simulink library "rov_design_analysis"  (Simulink 6.0)
settings: Solver=ode45  SolverMode=SingleTasking  StartTime=0.0  StopTime=10.0  RelTol=1e-3
undefined symbols (not defined in the file or in its folder): amp, At, B, Bt, Ct, cycles, D, den, DL, Do, DQ, DQL, freq, frtest, I, L, m, M, Ma, magnitude, MaU, Mt, nmiss, num, phase, rg, sigbuilder_block, slcm, T, W, xb, xg, Xudot, yb, yg, Yvdot, zb, zg, Zwdot
libraries: simulink_extras x32, simulink x27, rov_design_analysis x15, marine_gnc x10, dspmtrx2 x6, dspstat3 x4
(part 8 of 9)

== system rov_design_analysis/ROV Controller /Nonlinear-Sliding-Mode Cascaded  Controller - 6 DoF/Body-fixed to Earth_fixed Transformation3/Transformation matrix T/Row3 of R ==
  translational body velocity : Inport  Port=1  LatchInput=off
  angular position : Inport  Port=2  LatchInput=off
  -cZ.sX+sY.sZ.cX : Fcn  Expr=-cos(u[3])*sin(u[1]) + sin(u[2])*sin(u[3])*cos(u[1])
  Dot Product1 : Subsystem  mask(Dot Product){}
      mask help:
      | Inner (dot) product.
      | y=sum(u1.*u2)
      mask init:
      | t=(0:.1:2*pi)';
      | x=cos(t);
      | y=sin(t);
      mask Help: Computes the inner (dot) product of the inputs: sum(u1.*u2).  The inputs are vectors of the same length. Output is a scalar.
      mask Display: plot(0,0,1,1,x*[0.025 0.07]+0.5,y*[0.025 0.07]+0.5)
  Mux1 : Mux  Inputs=3
  cY.cX : Fcn  Expr=cos(u[2])*cos(u[1])
  sZ.sX+cZ.cX.sY : Fcn  Expr=sin(u[3])*sin(u[1]) + cos(u[3])*cos(u[1])*sin(u[2])
  translational earth velocity (row 3) : Outport  InitialOutput=0
  wires:
  Dot Product1/1(out_1) -> translational earth velocity (row 3)/1
  translational body velocity/1 -> Dot Product1/2(in_2)
  Mux1/1 -> Dot Product1/1(in_1)
  cY.cX/1 -> Mux1/3
  -cZ.sX+sY.sZ.cX/1 -> Mux1/2
  sZ.sX+cZ.cX.sY/1 -> Mux1/1
  angular position/1 -> cY.cX/1, -cZ.sX+sY.sZ.cX/1, sZ.sX+cZ.cX.sY/1

== system rov_design_analysis/ROV Controller /P-Decoupled  Cascaded loop Controller  - 6 DoF/Body-fixed to Earth_fixed Transformation1/Transformation matrix R/Row1 of T ==
  angular body  velocity : Inport  Port=1  LatchInput=off
  angular position : Inport  Port=2  LatchInput=off
  0 : Fcn  Expr=0
  1 : Fcn  Expr=1
  2 : Fcn  Expr=0
  Dot Product1 : Subsystem  mask(Dot Product){}
      mask help:
      | Inner (dot) product.
      | y=sum(u1.*u2)
      mask init:
      | t=(0:.1:2*pi)';
      | x=cos(t);
      | y=sin(t);
      mask Help: Computes the inner (dot) product of the inputs: sum(u1.*u2).  The inputs are vectors of the same length. Output is a scalar.
      mask Display: plot(0,0,1,1,x*[0.025 0.07]+0.5,y*[0.025 0.07]+0.5)
  Mux1 : Mux  Inputs=3
  angular earth velocity (row 1) : Outport  InitialOutput=0
  wires:
  angular position/1 -> 1/1, 0/1, 2/1
  1/1 -> Mux1/1
  0/1 -> Mux1/2
  2/1 -> Mux1/3
  Mux1/1 -> Dot Product1/1(in_1)
  angular body  velocity/1 -> Dot Product1/2(in_2)
  Dot Product1/1(out_1) -> angular earth velocity (row 1)/1

== system rov_design_analysis/ROV Controller /P-Decoupled  Cascaded loop Controller  - 6 DoF/Body-fixed to Earth_fixed Transformation1/Transformation matrix R/Row2 of T ==
  "angular body velocity " : Inport  Port=1  LatchInput=off
  angular position : Inport  Port=2  LatchInput=off
  Dot Product1 : Subsystem  mask(Dot Product){}
      mask help:
      | Inner (dot) product.
      | y=sum(u1.*u2)
      mask init:
      | t=(0:.1:2*pi)';
      | x=cos(t);
      | y=sin(t);
      mask Help: Computes the inner (dot) product of the inputs: sum(u1.*u2).  The inputs are vectors of the same length. Output is a scalar.
      mask Display: plot(0,0,1,1,x*[0.025 0.07]+0.5,y*[0.025 0.07]+0.5)
  Mux1 : Mux  Inputs=3
  cX : Fcn  Expr=cos(u[1])
  sX.tY : Fcn  Expr=sin(u[1])*tan(u[2])
  sX/cY : Fcn  Expr=sin(u[1])/cos(u[2])
  angular earth velocity (row 2) : Outport  InitialOutput=0
  wires:
  angular position/1 -> sX.tY/1, cX/1, sX/cY/1
  sX.tY/1 -> Mux1/1
  cX/1 -> Mux1/2
  sX/cY/1 -> Mux1/3
  Mux1/1 -> Dot Product1/1(in_1)
  "angular body velocity "/1 -> Dot Product1/2(in_2)
  Dot Product1/1(out_1) -> angular earth velocity (row 2)/1

== system rov_design_analysis/ROV Controller /P-Decoupled  Cascaded loop Controller  - 6 DoF/Body-fixed to Earth_fixed Transformation1/Transformation matrix R/Row3 of T ==
  "angular body velocity " : Inport  Port=1  LatchInput=off
  angular position : Inport  Port=2  LatchInput=off
  -sX : Fcn  Expr=-sin(u[1])
  Dot Product1 : Subsystem  mask(Dot Product){}
      mask help:
      | Inner (dot) product.
      | y=sum(u1.*u2)
      mask init:
      | t=(0:.1:2*pi)';
      | x=cos(t);
      | y=sin(t);
      mask Help: Computes the inner (dot) product of the inputs: sum(u1.*u2).  The inputs are vectors of the same length. Output is a scalar.
      mask Display: plot(0,0,1,1,x*[0.025 0.07]+0.5,y*[0.025 0.07]+0.5)
  Mux1 : Mux  Inputs=3
  cX.tY : Fcn  Expr=cos(u[1])*tan(u[2])
  cX/cY : Fcn  Expr=cos(u[1])/cos(u[2])
  angular earth velocity (row 3) : Outport  InitialOutput=0
  wires:
  angular position/1 -> cX.tY/1, -sX/1, cX/cY/1
  cX.tY/1 -> Mux1/1
  -sX/1 -> Mux1/2
  cX/cY/1 -> Mux1/3
  Mux1/1 -> Dot Product1/1(in_1)
  "angular body velocity "/1 -> Dot Product1/2(in_2)
  Dot Product1/1(out_1) -> angular earth velocity (row 3)/1

== system rov_design_analysis/ROV Controller /P-Decoupled  Cascaded loop Controller  - 6 DoF/Body-fixed to Earth_fixed Transformation1/Transformation matrix T/Row1 of R ==
  translational body velocity : Inport  Port=1  LatchInput=off
  angular position : Inport  Port=2  LatchInput=off
  -sY : Fcn  Expr=-sin(u[2])
  Dot Product : Subsystem  mask(Dot Product){}
      mask help:
      | Inner (dot) product.
      | y=sum(u1.*u2)
      mask init:
      | t=(0:.1:2*pi)';
      | x=cos(t);
      | y=sin(t);
      mask Help: Computes the inner (dot) product of the inputs: sum(u1.*u2).  The inputs are vectors of the same length. Output is a scalar.
      mask Display: plot(0,0,1,1,x*[0.025 0.07]+0.5,y*[0.025 0.07]+0.5)
  Mux : Mux  Inputs=3
  cY.cZ : Fcn  Expr=cos(u[3]) * cos(u[2])
  cY.sZ : Fcn  Expr=sin(u[3]) * cos(u[2])
  translational earth velocity (row 1) : Outport  InitialOutput=0
  wires:
  angular position/1 -> cY.cZ/1, cY.sZ/1, -sY/1
  cY.cZ/1 -> Mux/1
  cY.sZ/1 -> Mux/2
  -sY/1 -> Mux/3
  Mux/1 -> Dot Product/1(in_1)
  translational body velocity/1 -> Dot Product/2(in_2)
  Dot Product/1(out_1) -> translational earth velocity (row 1)/1

== system rov_design_analysis/ROV Controller /P-Decoupled  Cascaded loop Controller  - 6 DoF/Body-fixed to Earth_fixed Transformation1/Transformation matrix T/Row2 of R ==
  translational body velocity : Inport  Port=1  LatchInput=off
  angular position : Inport  Port=2  LatchInput=off
  -sZ.cX+cZ.sY.sX : Fcn  Expr=-sin(u[3])*cos(u[1]) + cos(u[3])*sin(u[2])*sin(u[1])
  Dot Product1 : Subsystem  mask(Dot Product){}
      mask help:
      | Inner (dot) product.
      | y=sum(u1.*u2)
      mask init:
      | t=(0:.1:2*pi)';
      | x=cos(t);
      | y=sin(t);
      mask Help: Computes the inner (dot) product of the inputs: sum(u1.*u2).  The inputs are vectors of the same length. Output is a scalar.
      mask Display: plot(0,0,1,1,x*[0.025 0.07]+0.5,y*[0.025 0.07]+0.5)
  Mux1 : Mux  Inputs=3
  cY.sX : Fcn  Expr=cos(u[2])*sin(u[1])
  cZ.cX+sX.sY.sZ : Fcn  Expr=cos(u[3])*cos(u[1]) + sin(u[1])*sin(u[2])*sin(u[3])
  translational earth velocity (row 2) : Outport  InitialOutput=0
  wires:
  angular position/1 -> -sZ.cX+cZ.sY.sX/1, cZ.cX+sX.sY.sZ/1, cY.sX/1
  -sZ.cX+cZ.sY.sX/1 -> Mux1/1
  cZ.cX+sX.sY.sZ/1 -> Mux1/2
  cY.sX/1 -> Mux1/3
  Mux1/1 -> Dot Product1/1(in_1)
  translational body velocity/1 -> Dot Product1/2(in_2)
  Dot Product1/1(out_1) -> translational earth velocity (row 2)/1

== system rov_design_analysis/ROV Controller /P-Decoupled  Cascaded loop Controller  - 6 DoF/Body-fixed to Earth_fixed Transformation1/Transformation matrix T/Row3 of R ==
  translational body velocity : Inport  Port=1  LatchInput=off
  angular position : Inport  Port=2  LatchInput=off
  -cZ.sX+sY.sZ.cX : Fcn  Expr=-cos(u[3])*sin(u[1]) + sin(u[2])*sin(u[3])*cos(u[1])
  Dot Product1 : Subsystem  mask(Dot Product){}
      mask help:
      | Inner (dot) product.
      | y=sum(u1.*u2)
      mask init:
      | t=(0:.1:2*pi)';
      | x=cos(t);
      | y=sin(t);
      mask Help: Computes the inner (dot) product of the inputs: sum(u1.*u2).  The inputs are vectors of the same length. Output is a scalar.
      mask Display: plot(0,0,1,1,x*[0.025 0.07]+0.5,y*[0.025 0.07]+0.5)
  Mux1 : Mux  Inputs=3
  cY.cX : Fcn  Expr=cos(u[2])*cos(u[1])
  sZ.sX+cZ.cX.sY : Fcn  Expr=sin(u[3])*sin(u[1]) + cos(u[3])*cos(u[1])*sin(u[2])
  translational earth velocity (row 3) : Outport  InitialOutput=0
  wires:
  angular position/1 -> sZ.sX+cZ.cX.sY/1, -cZ.sX+sY.sZ.cX/1, cY.cX/1
  sZ.sX+cZ.cX.sY/1 -> Mux1/1
  -cZ.sX+sY.sZ.cX/1 -> Mux1/2
  cY.cX/1 -> Mux1/3
  Mux1/1 -> Dot Product1/1(in_1)
  translational body velocity/1 -> Dot Product1/2(in_2)
  Dot Product1/1(out_1) -> translational earth velocity (row 3)/1

== system rov_design_analysis/ROV Controller /P-Decoupled  Cascaded loop Controller  - 6 DoF/Body-fixed to Earth_fixed Transformation3/Transformation matrix R/Row1 of T ==
  angular body  velocity : Inport  Port=1  LatchInput=off
  angular position : Inport  Port=2  LatchInput=off
  0 : Fcn  Expr=0
  1 : Fcn  Expr=1
  2 : Fcn  Expr=0
  Dot Product1 : Subsystem  mask(Dot Product){}
      mask help:
      | Inner (dot) product.
      | y=sum(u1.*u2)
      mask init:
      | t=(0:.1:2*pi)';
      | x=cos(t);
      | y=sin(t);
      mask Help: Computes the inner (dot) product of the inputs: sum(u1.*u2).  The inputs are vectors of the same length. Output is a scalar.
      mask Display: plot(0,0,1,1,x*[0.025 0.07]+0.5,y*[0.025 0.07]+0.5)
  Mux1 : Mux  Inputs=3
  angular earth velocity (row 1) : Outport  InitialOutput=0
  wires:
  Dot Product1/1(out_1) -> angular earth velocity (row 1)/1
  angular body  velocity/1 -> Dot Product1/2(in_2)
  Mux1/1 -> Dot Product1/1(in_1)
  2/1 -> Mux1/3
  0/1 -> Mux1/2
  1/1 -> Mux1/1
  angular position/1 -> 2/1, 0/1, 1/1

== system rov_design_analysis/ROV Controller /P-Decoupled  Cascaded loop Controller  - 6 DoF/Body-fixed to Earth_fixed Transformation3/Transformation matrix R/Row2 of T ==
  "angular body velocity " : Inport  Port=1  LatchInput=off
  angular position : Inport  Port=2  LatchInput=off
  Dot Product1 : Subsystem  mask(Dot Product){}
      mask help:
      | Inner (dot) product.
      | y=sum(u1.*u2)
      mask init:
      | t=(0:.1:2*pi)';
      | x=cos(t);
      | y=sin(t);
      mask Help: Computes the inner (dot) product of the inputs: sum(u1.*u2).  The inputs are vectors of the same length. Output is a scalar.
      mask Display: plot(0,0,1,1,x*[0.025 0.07]+0.5,y*[0.025 0.07]+0.5)
  Mux1 : Mux  Inputs=3
  cX : Fcn  Expr=cos(u[1])
  sX.tY : Fcn  Expr=sin(u[1])*tan(u[2])
  sX/cY : Fcn  Expr=sin(u[1])/cos(u[2])
  angular earth velocity (row 2) : Outport  InitialOutput=0
  wires:
  Dot Product1/1(out_1) -> angular earth velocity (row 2)/1
  "angular body velocity "/1 -> Dot Product1/2(in_2)
  Mux1/1 -> Dot Product1/1(in_1)
  sX/cY/1 -> Mux1/3
  cX/1 -> Mux1/2
  sX.tY/1 -> Mux1/1
  angular position/1 -> sX/cY/1, cX/1, sX.tY/1

== system rov_design_analysis/ROV Controller /P-Decoupled  Cascaded loop Controller  - 6 DoF/Body-fixed to Earth_fixed Transformation3/Transformation matrix R/Row3 of T ==
  "angular body velocity " : Inport  Port=1  LatchInput=off
  angular position : Inport  Port=2  LatchInput=off
  -sX : Fcn  Expr=-sin(u[1])
  Dot Product1 : Subsystem  mask(Dot Product){}
      mask help:
      | Inner (dot) product.
      | y=sum(u1.*u2)
      mask init:
      | t=(0:.1:2*pi)';
      | x=cos(t);
      | y=sin(t);
      mask Help: Computes the inner (dot) product of the inputs: sum(u1.*u2).  The inputs are vectors of the same length. Output is a scalar.
      mask Display: plot(0,0,1,1,x*[0.025 0.07]+0.5,y*[0.025 0.07]+0.5)
  Mux1 : Mux  Inputs=3
  cX.tY : Fcn  Expr=cos(u[1])*tan(u[2])
  cX/cY : Fcn  Expr=cos(u[1])/cos(u[2])
  angular earth velocity (row 3) : Outport  InitialOutput=0
  wires:
  Dot Product1/1(out_1) -> angular earth velocity (row 3)/1
  "angular body velocity "/1 -> Dot Product1/2(in_2)
  Mux1/1 -> Dot Product1/1(in_1)
  cX/cY/1 -> Mux1/3
  -sX/1 -> Mux1/2
  cX.tY/1 -> Mux1/1
  angular position/1 -> cX/cY/1, -sX/1, cX.tY/1

== system rov_design_analysis/ROV Controller /P-Decoupled  Cascaded loop Controller  - 6 DoF/Body-fixed to Earth_fixed Transformation3/Transformation matrix T/Row1 of R ==
  translational body velocity : Inport  Port=1  LatchInput=off
  angular position : Inport  Port=2  LatchInput=off
  -sY : Fcn  Expr=-sin(u[2])
  Dot Product : Subsystem  mask(Dot Product){}
      mask help:
      | Inner (dot) product.
      | y=sum(u1.*u2)
      mask init:
      | t=(0:.1:2*pi)';
      | x=cos(t);
      | y=sin(t);
      mask Help: Computes the inner (dot) product of the inputs: sum(u1.*u2).  The inputs are vectors of the same length. Output is a scalar.
      mask Display: plot(0,0,1,1,x*[0.025 0.07]+0.5,y*[0.025 0.07]+0.5)
  Mux : Mux  Inputs=3
  cY.cZ : Fcn  Expr=cos(u[3]) * cos(u[2])
  cY.sZ : Fcn  Expr=sin(u[3]) * cos(u[2])
  translational earth velocity (row 1) : Outport  InitialOutput=0
  wires:
  Dot Product/1(out_1) -> translational earth velocity (row 1)/1
  translational body velocity/1 -> Dot Product/2(in_2)
  Mux/1 -> Dot Product/1(in_1)
  -sY/1 -> Mux/3
  cY.sZ/1 -> Mux/2
  cY.cZ/1 -> Mux/1
  angular position/1 -> -sY/1, cY.sZ/1, cY.cZ/1

== system rov_design_analysis/ROV Controller /P-Decoupled  Cascaded loop Controller  - 6 DoF/Body-fixed to Earth_fixed Transformation3/Transformation matrix T/Row2 of R ==
  translational body velocity : Inport  Port=1  LatchInput=off
  angular position : Inport  Port=2  LatchInput=off
  -sZ.cX+cZ.sY.sX : Fcn  Expr=-sin(u[3])*cos(u[1]) + cos(u[3])*sin(u[2])*sin(u[1])
  Dot Product1 : Subsystem  mask(Dot Product){}
      mask help:
      | Inner (dot) product.
      | y=sum(u1.*u2)
      mask init:
      | t=(0:.1:2*pi)';
      | x=cos(t);
      | y=sin(t);
      mask Help: Computes the inner (dot) product of the inputs: sum(u1.*u2).  The inputs are vectors of the same length. Output is a scalar.
      mask Display: plot(0,0,1,1,x*[0.025 0.07]+0.5,y*[0.025 0.07]+0.5)
  Mux1 : Mux  Inputs=3
  cY.sX : Fcn  Expr=cos(u[2])*sin(u[1])
  cZ.cX+sX.sY.sZ : Fcn  Expr=cos(u[3])*cos(u[1]) + sin(u[1])*sin(u[2])*sin(u[3])
  translational earth velocity (row 2) : Outport  InitialOutput=0
  wires:
  Dot Product1/1(out_1) -> translational earth velocity (row 2)/1
  translational body velocity/1 -> Dot Product1/2(in_2)
  Mux1/1 -> Dot Product1/1(in_1)
  cY.sX/1 -> Mux1/3
  cZ.cX+sX.sY.sZ/1 -> Mux1/2
  -sZ.cX+cZ.sY.sX/1 -> Mux1/1
  angular position/1 -> cY.sX/1, cZ.cX+sX.sY.sZ/1, -sZ.cX+cZ.sY.sX/1

== system rov_design_analysis/ROV Controller /P-Decoupled  Cascaded loop Controller  - 6 DoF/Body-fixed to Earth_fixed Transformation3/Transformation matrix T/Row3 of R ==
  translational body velocity : Inport  Port=1  LatchInput=off
  angular position : Inport  Port=2  LatchInput=off
  -cZ.sX+sY.sZ.cX : Fcn  Expr=-cos(u[3])*sin(u[1]) + sin(u[2])*sin(u[3])*cos(u[1])
  Dot Product1 : Subsystem  mask(Dot Product){}
      mask help:
      | Inner (dot) product.
      | y=sum(u1.*u2)
      mask init:
      | t=(0:.1:2*pi)';
      | x=cos(t);
      | y=sin(t);
      mask Help: Computes the inner (dot) product of the inputs: sum(u1.*u2).  The inputs are vectors of the same length. Output is a scalar.
      mask Display: plot(0,0,1,1,x*[0.025 0.07]+0.5,y*[0.025 0.07]+0.5)
  Mux1 : Mux  Inputs=3
  cY.cX : Fcn  Expr=cos(u[2])*cos(u[1])
  sZ.sX+cZ.cX.sY : Fcn  Expr=sin(u[3])*sin(u[1]) + cos(u[3])*cos(u[1])*sin(u[2])
  translational earth velocity (row 3) : Outport  InitialOutput=0
  wires:
  Dot Product1/1(out_1) -> translational earth velocity (row 3)/1
  translational body velocity/1 -> Dot Product1/2(in_2)
  Mux1/1 -> Dot Product1/1(in_1)
  cY.cX/1 -> Mux1/3
  -cZ.sX+sY.sZ.cX/1 -> Mux1/2
  sZ.sX+cZ.cX.sY/1 -> Mux1/1
  angular position/1 -> cY.cX/1, -cZ.sX+sY.sZ.cX/1, sZ.sX+cZ.cX.sY/1

== system rov_design_analysis/ROV Controller /P-Decoupled  Single loop Controller - 6 DoF /Body-fixed to Earth_fixed Transformation1/Transformation matrix R/Row1 of T ==
  angular body  velocity : Inport  Port=1  LatchInput=off
  angular position : Inport  Port=2  LatchInput=off
  0 : Fcn  Expr=0
  1 : Fcn  Expr=1
  2 : Fcn  Expr=0
  Dot Product1 : Subsystem  mask(Dot Product){}
      mask help:
      | Inner (dot) product.
      | y=sum(u1.*u2)
      mask init:
      | t=(0:.1:2*pi)';
      | x=cos(t);
      | y=sin(t);
      mask Help: Computes the inner (dot) product of the inputs: sum(u1.*u2).  The inputs are vectors of the same length. Output is a scalar.
      mask Display: plot(0,0,1,1,x*[0.025 0.07]+0.5,y*[0.025 0.07]+0.5)
  Mux1 : Mux  Inputs=3
  angular earth velocity (row 1) : Outport  InitialOutput=0
  wires:
  Dot Product1/1(out_1) -> angular earth velocity (row 1)/1
  angular body  velocity/1 -> Dot Product1/2(in_2)
  Mux1/1 -> Dot Product1/1(in_1)
  2/1 -> Mux1/3
  0/1 -> Mux1/2
  1/1 -> Mux1/1
  angular position/1 -> 2/1, 0/1, 1/1

== system rov_design_analysis/ROV Controller /P-Decoupled  Single loop Controller - 6 DoF /Body-fixed to Earth_fixed Transformation1/Transformation matrix R/Row2 of T ==
  "angular body velocity " : Inport  Port=1  LatchInput=off
  angular position : Inport  Port=2  LatchInput=off
  Dot Product1 : Subsystem  mask(Dot Product){}
      mask help:
      | Inner (dot) product.
      | y=sum(u1.*u2)
      mask init:
      | t=(0:.1:2*pi)';
      | x=cos(t);
      | y=sin(t);
      mask Help: Computes the inner (dot) product of the inputs: sum(u1.*u2).  The inputs are vectors of the same length. Output is a scalar.
      mask Display: plot(0,0,1,1,x*[0.025 0.07]+0.5,y*[0.025 0.07]+0.5)
  Mux1 : Mux  Inputs=3
  cX : Fcn  Expr=cos(u[1])
  sX.tY : Fcn  Expr=sin(u[1])*tan(u[2])
  sX/cY : Fcn  Expr=sin(u[1])/cos(u[2])
  angular earth velocity (row 2) : Outport  InitialOutput=0
  wires:
  Dot Product1/1(out_1) -> angular earth velocity (row 2)/1
  "angular body velocity "/1 -> Dot Product1/2(in_2)
  Mux1/1 -> Dot Product1/1(in_1)
  sX/cY/1 -> Mux1/3
  cX/1 -> Mux1/2
  sX.tY/1 -> Mux1/1
  angular position/1 -> sX/cY/1, cX/1, sX.tY/1

== system rov_design_analysis/ROV Controller /P-Decoupled  Single loop Controller - 6 DoF /Body-fixed to Earth_fixed Transformation1/Transformation matrix R/Row3 of T ==
  "angular body velocity " : Inport  Port=1  LatchInput=off
  angular position : Inport  Port=2  LatchInput=off
  -sX : Fcn  Expr=-sin(u[1])
  Dot Product1 : Subsystem  mask(Dot Product){}
      mask help:
      | Inner (dot) product.
      | y=sum(u1.*u2)
      mask init:
      | t=(0:.1:2*pi)';
      | x=cos(t);
      | y=sin(t);
      mask Help: Computes the inner (dot) product of the inputs: sum(u1.*u2).  The inputs are vectors of the same length. Output is a scalar.
      mask Display: plot(0,0,1,1,x*[0.025 0.07]+0.5,y*[0.025 0.07]+0.5)
  Mux1 : Mux  Inputs=3
  cX.tY : Fcn  Expr=cos(u[1])*tan(u[2])
  cX/cY : Fcn  Expr=cos(u[1])/cos(u[2])
  angular earth velocity (row 3) : Outport  InitialOutput=0
  wires:
  Dot Product1/1(out_1) -> angular earth velocity (row 3)/1
  "angular body velocity "/1 -> Dot Product1/2(in_2)
  Mux1/1 -> Dot Product1/1(in_1)
  cX/cY/1 -> Mux1/3
  -sX/1 -> Mux1/2
  cX.tY/1 -> Mux1/1
  angular position/1 -> cX/cY/1, -sX/1, cX.tY/1

== system rov_design_analysis/ROV Controller /P-Decoupled  Single loop Controller - 6 DoF /Body-fixed to Earth_fixed Transformation1/Transformation matrix T/Row1 of R ==
  translational body velocity : Inport  Port=1  LatchInput=off
  angular position : Inport  Port=2  LatchInput=off
  -sY : Fcn  Expr=-sin(u[2])
  Dot Product : Subsystem  mask(Dot Product){}
      mask help:
      | Inner (dot) product.
      | y=sum(u1.*u2)
      mask init:
      | t=(0:.1:2*pi)';
      | x=cos(t);
      | y=sin(t);
      mask Help: Computes the inner (dot) product of the inputs: sum(u1.*u2).  The inputs are vectors of the same length. Output is a scalar.
      mask Display: plot(0,0,1,1,x*[0.025 0.07]+0.5,y*[0.025 0.07]+0.5)
  Mux : Mux  Inputs=3
  cY.cZ : Fcn  Expr=cos(u[3]) * cos(u[2])
  cY.sZ : Fcn  Expr=sin(u[3]) * cos(u[2])
  translational earth velocity (row 1) : Outport  InitialOutput=0
  wires:
  Dot Product/1(out_1) -> translational earth velocity (row 1)/1
  translational body velocity/1 -> Dot Product/2(in_2)
  Mux/1 -> Dot Product/1(in_1)
  -sY/1 -> Mux/3
  cY.sZ/1 -> Mux/2
  cY.cZ/1 -> Mux/1
  angular position/1 -> -sY/1, cY.sZ/1, cY.cZ/1

== system rov_design_analysis/ROV Controller /P-Decoupled  Single loop Controller - 6 DoF /Body-fixed to Earth_fixed Transformation1/Transformation matrix T/Row2 of R ==
  translational body velocity : Inport  Port=1  LatchInput=off
  angular position : Inport  Port=2  LatchInput=off
  -sZ.cX+cZ.sY.sX : Fcn  Expr=-sin(u[3])*cos(u[1]) + cos(u[3])*sin(u[2])*sin(u[1])
  Dot Product1 : Subsystem  mask(Dot Product){}
      mask help:
      | Inner (dot) product.
      | y=sum(u1.*u2)
      mask init:
      | t=(0:.1:2*pi)';
      | x=cos(t);
      | y=sin(t);
      mask Help: Computes the inner (dot) product of the inputs: sum(u1.*u2).  The inputs are vectors of the same length. Output is a scalar.
      mask Display: plot(0,0,1,1,x*[0.025 0.07]+0.5,y*[0.025 0.07]+0.5)
  Mux1 : Mux  Inputs=3
  cY.sX : Fcn  Expr=cos(u[2])*sin(u[1])
  cZ.cX+sX.sY.sZ : Fcn  Expr=cos(u[3])*cos(u[1]) + sin(u[1])*sin(u[2])*sin(u[3])
  translational earth velocity (row 2) : Outport  InitialOutput=0
  wires:
  Dot Product1/1(out_1) -> translational earth velocity (row 2)/1
  translational body velocity/1 -> Dot Product1/2(in_2)
  Mux1/1 -> Dot Product1/1(in_1)
  cY.sX/1 -> Mux1/3
  cZ.cX+sX.sY.sZ/1 -> Mux1/2
  -sZ.cX+cZ.sY.sX/1 -> Mux1/1
  angular position/1 -> cY.sX/1, cZ.cX+sX.sY.sZ/1, -sZ.cX+cZ.sY.sX/1

== system rov_design_analysis/ROV Controller /P-Decoupled  Single loop Controller - 6 DoF /Body-fixed to Earth_fixed Transformation1/Transformation matrix T/Row3 of R ==
  translational body velocity : Inport  Port=1  LatchInput=off
  angular position : Inport  Port=2  LatchInput=off
  -cZ.sX+sY.sZ.cX : Fcn  Expr=-cos(u[3])*sin(u[1]) + sin(u[2])*sin(u[3])*cos(u[1])
  Dot Product1 : Subsystem  mask(Dot Product){}
      mask help:
      | Inner (dot) product.
      | y=sum(u1.*u2)
      mask init:
      | t=(0:.1:2*pi)';
      | x=cos(t);
      | y=sin(t);
      mask Help: Computes the inner (dot) product of the inputs: sum(u1.*u2).  The inputs are vectors of the same length. Output is a scalar.
      mask Display: plot(0,0,1,1,x*[0.025 0.07]+0.5,y*[0.025 0.07]+0.5)
  Mux1 : Mux  Inputs=3
  cY.cX : Fcn  Expr=cos(u[2])*cos(u[1])
  sZ.sX+cZ.cX.sY : Fcn  Expr=sin(u[3])*sin(u[1]) + cos(u[3])*cos(u[1])*sin(u[2])
  translational earth velocity (row 3) : Outport  InitialOutput=0
  wires:
  Dot Product1/1(out_1) -> translational earth velocity (row 3)/1
  translational body velocity/1 -> Dot Product1/2(in_2)
  Mux1/1 -> Dot Product1/1(in_1)
  cY.cX/1 -> Mux1/3
  -cZ.sX+sY.sZ.cX/1 -> Mux1/2
  sZ.sX+cZ.cX.sY/1 -> Mux1/1
  angular position/1 -> cY.cX/1, -cZ.sX+sY.sZ.cX/1, sZ.sX+cZ.cX.sY/1

== system rov_design_analysis/ROV Controller /P-Decoupled  Single loop Controller - 6 DoF /Body-fixed to Earth_fixed Transformation3/Transformation matrix R/Row1 of T ==
  angular body  velocity : Inport  Port=1  LatchInput=off
  angular position : Inport  Port=2  LatchInput=off
  0 : Fcn  Expr=0
  1 : Fcn  Expr=1
  2 : Fcn  Expr=0
  Dot Product1 : Subsystem  mask(Dot Product){}
      mask help:
      | Inner (dot) product.
      | y=sum(u1.*u2)
      mask init:
      | t=(0:.1:2*pi)';
      | x=cos(t);
      | y=sin(t);
      mask Help: Computes the inner (dot) product of the inputs: sum(u1.*u2).  The inputs are vectors of the same length. Output is a scalar.
      mask Display: plot(0,0,1,1,x*[0.025 0.07]+0.5,y*[0.025 0.07]+0.5)
  Mux1 : Mux  Inputs=3
  angular earth velocity (row 1) : Outport  InitialOutput=0
  wires:
  angular position/1 -> 1/1, 0/1, 2/1
  1/1 -> Mux1/1
  0/1 -> Mux1/2
  2/1 -> Mux1/3
  Mux1/1 -> Dot Product1/1(in_1)
  angular body  velocity/1 -> Dot Product1/2(in_2)
  Dot Product1/1(out_1) -> angular earth velocity (row 1)/1

== system rov_design_analysis/ROV Controller /P-Decoupled  Single loop Controller - 6 DoF /Body-fixed to Earth_fixed Transformation3/Transformation matrix R/Row2 of T ==
  "angular body velocity " : Inport  Port=1  LatchInput=off
  angular position : Inport  Port=2  LatchInput=off
  Dot Product1 : Subsystem  mask(Dot Product){}
      mask help:
      | Inner (dot) product.
      | y=sum(u1.*u2)
      mask init:
      | t=(0:.1:2*pi)';
      | x=cos(t);
      | y=sin(t);
      mask Help: Computes the inner (dot) product of the inputs: sum(u1.*u2).  The inputs are vectors of the same length. Output is a scalar.
      mask Display: plot(0,0,1,1,x*[0.025 0.07]+0.5,y*[0.025 0.07]+0.5)
  Mux1 : Mux  Inputs=3
  cX : Fcn  Expr=cos(u[1])
  sX.tY : Fcn  Expr=sin(u[1])*tan(u[2])
  sX/cY : Fcn  Expr=sin(u[1])/cos(u[2])
  angular earth velocity (row 2) : Outport  InitialOutput=0
  wires:
  angular position/1 -> sX.tY/1, cX/1, sX/cY/1
  sX.tY/1 -> Mux1/1
  cX/1 -> Mux1/2
  sX/cY/1 -> Mux1/3
  Mux1/1 -> Dot Product1/1(in_1)
  "angular body velocity "/1 -> Dot Product1/2(in_2)
  Dot Product1/1(out_1) -> angular earth velocity (row 2)/1

== system rov_design_analysis/ROV Controller /P-Decoupled  Single loop Controller - 6 DoF /Body-fixed to Earth_fixed Transformation3/Transformation matrix R/Row3 of T ==
  "angular body velocity " : Inport  Port=1  LatchInput=off
  angular position : Inport  Port=2  LatchInput=off
  -sX : Fcn  Expr=-sin(u[1])
  Dot Product1 : Subsystem  mask(Dot Product){}
      mask help:
      | Inner (dot) product.
      | y=sum(u1.*u2)
      mask init:
      | t=(0:.1:2*pi)';
      | x=cos(t);
      | y=sin(t);
      mask Help: Computes the inner (dot) product of the inputs: sum(u1.*u2).  The inputs are vectors of the same length. Output is a scalar.
      mask Display: plot(0,0,1,1,x*[0.025 0.07]+0.5,y*[0.025 0.07]+0.5)
  Mux1 : Mux  Inputs=3
  cX.tY : Fcn  Expr=cos(u[1])*tan(u[2])
  cX/cY : Fcn  Expr=cos(u[1])/cos(u[2])
  angular earth velocity (row 3) : Outport  InitialOutput=0
  wires:
  angular position/1 -> cX.tY/1, -sX/1, cX/cY/1
  cX.tY/1 -> Mux1/1
  -sX/1 -> Mux1/2
  cX/cY/1 -> Mux1/3
  Mux1/1 -> Dot Product1/1(in_1)
  "angular body velocity "/1 -> Dot Product1/2(in_2)
  Dot Product1/1(out_1) -> angular earth velocity (row 3)/1

== system rov_design_analysis/ROV Controller /P-Decoupled  Single loop Controller - 6 DoF /Body-fixed to Earth_fixed Transformation3/Transformation matrix T/Row1 of R ==
  translational body velocity : Inport  Port=1  LatchInput=off
  angular position : Inport  Port=2  LatchInput=off
  -sY : Fcn  Expr=-sin(u[2])
  Dot Product : Subsystem  mask(Dot Product){}
      mask help:
      | Inner (dot) product.
      | y=sum(u1.*u2)
      mask init:
      | t=(0:.1:2*pi)';
      | x=cos(t);
      | y=sin(t);
      mask Help: Computes the inner (dot) product of the inputs: sum(u1.*u2).  The inputs are vectors of the same length. Output is a scalar.
      mask Display: plot(0,0,1,1,x*[0.025 0.07]+0.5,y*[0.025 0.07]+0.5)
  Mux : Mux  Inputs=3
  cY.cZ : Fcn  Expr=cos(u[3]) * cos(u[2])
  cY.sZ : Fcn  Expr=sin(u[3]) * cos(u[2])
  translational earth velocity (row 1) : Outport  InitialOutput=0
  wires:
  angular position/1 -> cY.cZ/1, cY.sZ/1, -sY/1
  cY.cZ/1 -> Mux/1
  cY.sZ/1 -> Mux/2
  -sY/1 -> Mux/3
  Mux/1 -> Dot Product/1(in_1)
  translational body velocity/1 -> Dot Product/2(in_2)
  Dot Product/1(out_1) -> translational earth velocity (row 1)/1

== system rov_design_analysis/ROV Controller /P-Decoupled  Single loop Controller - 6 DoF /Body-fixed to Earth_fixed Transformation3/Transformation matrix T/Row2 of R ==
  translational body velocity : Inport  Port=1  LatchInput=off
  angular position : Inport  Port=2  LatchInput=off
  -sZ.cX+cZ.sY.sX : Fcn  Expr=-sin(u[3])*cos(u[1]) + cos(u[3])*sin(u[2])*sin(u[1])
  Dot Product1 : Subsystem  mask(Dot Product){}
      mask help:
      | Inner (dot) product.
      | y=sum(u1.*u2)
      mask init:
      | t=(0:.1:2*pi)';
      | x=cos(t);
      | y=sin(t);
      mask Help: Computes the inner (dot) product of the inputs: sum(u1.*u2).  The inputs are vectors of the same length. Output is a scalar.
      mask Display: plot(0,0,1,1,x*[0.025 0.07]+0.5,y*[0.025 0.07]+0.5)
  Mux1 : Mux  Inputs=3
  cY.sX : Fcn  Expr=cos(u[2])*sin(u[1])
  cZ.cX+sX.sY.sZ : Fcn  Expr=cos(u[3])*cos(u[1]) + sin(u[1])*sin(u[2])*sin(u[3])
  translational earth velocity (row 2) : Outport  InitialOutput=0
  wires:
  angular position/1 -> -sZ.cX+cZ.sY.sX/1, cZ.cX+sX.sY.sZ/1, cY.sX/1
  -sZ.cX+cZ.sY.sX/1 -> Mux1/1
  cZ.cX+sX.sY.sZ/1 -> Mux1/2
  cY.sX/1 -> Mux1/3
  Mux1/1 -> Dot Product1/1(in_1)
  translational body velocity/1 -> Dot Product1/2(in_2)
  Dot Product1/1(out_1) -> translational earth velocity (row 2)/1

== system rov_design_analysis/ROV Controller /P-Decoupled  Single loop Controller - 6 DoF /Body-fixed to Earth_fixed Transformation3/Transformation matrix T/Row3 of R ==
  translational body velocity : Inport  Port=1  LatchInput=off
  angular position : Inport  Port=2  LatchInput=off
  -cZ.sX+sY.sZ.cX : Fcn  Expr=-cos(u[3])*sin(u[1]) + sin(u[2])*sin(u[3])*cos(u[1])
  Dot Product1 : Subsystem  mask(Dot Product){}
      mask help:
      | Inner (dot) product.
      | y=sum(u1.*u2)
      mask init:
      | t=(0:.1:2*pi)';
      | x=cos(t);
      | y=sin(t);
      mask Help: Computes the inner (dot) product of the inputs: sum(u1.*u2).  The inputs are vectors of the same length. Output is a scalar.
      mask Display: plot(0,0,1,1,x*[0.025 0.07]+0.5,y*[0.025 0.07]+0.5)
  Mux1 : Mux  Inputs=3
  cY.cX : Fcn  Expr=cos(u[2])*cos(u[1])
  sZ.sX+cZ.cX.sY : Fcn  Expr=sin(u[3])*sin(u[1]) + cos(u[3])*cos(u[1])*sin(u[2])
  translational earth velocity (row 3) : Outport  InitialOutput=0
  wires:
  angular position/1 -> sZ.sX+cZ.cX.sY/1, -cZ.sX+sY.sZ.cX/1, cY.cX/1
  sZ.sX+cZ.cX.sY/1 -> Mux1/1
  -cZ.sX+sY.sZ.cX/1 -> Mux1/2
  cY.cX/1 -> Mux1/3
  Mux1/1 -> Dot Product1/1(in_1)
  translational body velocity/1 -> Dot Product1/2(in_2)
  Dot Product1/1(out_1) -> translational earth velocity (row 3)/1

== system rov_design_analysis/ROV Controller /Adaptive PD  Cascaded  Controller - 6 DoF/Body-fixed to Earth_fixed Transformation1/Transformation matrix R/Row1 of T/Dot Product1 ==
  in_1 : Inport  Port=1  LatchInput=off
  in_2 : Inport  Port=2  LatchInput=off
  Product : Product  SaturateOnIntegerOverflow=on  RndMeth=Zero  InputSameDT=on
  Sum : Sum  Inputs=+  SaturateOnIntegerOverflow=on  InputSameDT=on
  out_1 : Outport  InitialOutput=0
  wires:
  Sum/1 -> out_1/1
  Product/1 -> Sum/1
  in_1/1 -> Product/1
  in_2/1 -> Product/2

== system rov_design_analysis/ROV Controller /Adaptive PD  Cascaded  Controller - 6 DoF/Body-fixed to Earth_fixed Transformation1/Transformation matrix R/Row2 of T/Dot Product1 ==
  in_1 : Inport  Port=1  LatchInput=off
  in_2 : Inport  Port=2  LatchInput=off
  Product : Product  SaturateOnIntegerOverflow=on  RndMeth=Zero  InputSameDT=on
  Sum : Sum  Inputs=+  SaturateOnIntegerOverflow=on  InputSameDT=on
  out_1 : Outport  InitialOutput=0
  wires:
  Sum/1 -> out_1/1
  Product/1 -> Sum/1
  in_1/1 -> Product/1
  in_2/1 -> Product/2

== system rov_design_analysis/ROV Controller /Adaptive PD  Cascaded  Controller - 6 DoF/Body-fixed to Earth_fixed Transformation1/Transformation matrix R/Row3 of T/Dot Product1 ==
  in_1 : Inport  Port=1  LatchInput=off
  in_2 : Inport  Port=2  LatchInput=off
  Product : Product  SaturateOnIntegerOverflow=on  RndMeth=Zero  InputSameDT=on
  Sum : Sum  Inputs=+  SaturateOnIntegerOverflow=on  InputSameDT=on
  out_1 : Outport  InitialOutput=0
  wires:
  Sum/1 -> out_1/1
  Product/1 -> Sum/1
  in_1/1 -> Product/1
  in_2/1 -> Product/2

== system rov_design_analysis/ROV Controller /Adaptive PD  Cascaded  Controller - 6 DoF/Body-fixed to Earth_fixed Transformation1/Transformation matrix T/Row1 of R/Dot Product ==
  in_1 : Inport  Port=1  LatchInput=off
  in_2 : Inport  Port=2  LatchInput=off
  Product : Product  SaturateOnIntegerOverflow=on  RndMeth=Zero  InputSameDT=on
  Sum : Sum  Inputs=+  SaturateOnIntegerOverflow=on  InputSameDT=on
  out_1 : Outport  InitialOutput=0
  wires:
  Sum/1 -> out_1/1
  Product/1 -> Sum/1
  in_1/1 -> Product/1
  in_2/1 -> Product/2

== system rov_design_analysis/ROV Controller /Adaptive PD  Cascaded  Controller - 6 DoF/Body-fixed to Earth_fixed Transformation1/Transformation matrix T/Row2 of R/Dot Product1 ==
  in_1 : Inport  Port=1  LatchInput=off
  in_2 : Inport  Port=2  LatchInput=off
  Product : Product  SaturateOnIntegerOverflow=on  RndMeth=Zero  InputSameDT=on
  Sum : Sum  Inputs=+  SaturateOnIntegerOverflow=on  InputSameDT=on
  out_1 : Outport  InitialOutput=0
  wires:
  Sum/1 -> out_1/1
  Product/1 -> Sum/1
  in_1/1 -> Product/1
  in_2/1 -> Product/2

== system rov_design_analysis/ROV Controller /Adaptive PD  Cascaded  Controller - 6 DoF/Body-fixed to Earth_fixed Transformation1/Transformation matrix T/Row3 of R/Dot Product1 ==
  in_1 : Inport  Port=1  LatchInput=off
  in_2 : Inport  Port=2  LatchInput=off
  Product : Product  SaturateOnIntegerOverflow=on  RndMeth=Zero  InputSameDT=on
  Sum : Sum  Inputs=+  SaturateOnIntegerOverflow=on  InputSameDT=on
  out_1 : Outport  InitialOutput=0
  wires:
  Sum/1 -> out_1/1
  Product/1 -> Sum/1
  in_1/1 -> Product/1
  in_2/1 -> Product/2

== system rov_design_analysis/ROV Controller /Adaptive PD  Cascaded  Controller - 6 DoF/Body-fixed to Earth_fixed Transformation3/Transformation matrix R/Row1 of T/Dot Product1 ==
  in_1 : Inport  Port=1  LatchInput=off
  in_2 : Inport  Port=2  LatchInput=off
  Product : Product  SaturateOnIntegerOverflow=on  RndMeth=Zero  InputSameDT=on
  Sum : Sum  Inputs=+  SaturateOnIntegerOverflow=on  InputSameDT=on
  out_1 : Outport  InitialOutput=0
  wires:
  in_2/1 -> Product/2
  in_1/1 -> Product/1
  Product/1 -> Sum/1
  Sum/1 -> out_1/1

== system rov_design_analysis/ROV Controller /Adaptive PD  Cascaded  Controller - 6 DoF/Body-fixed to Earth_fixed Transformation3/Transformation matrix R/Row2 of T/Dot Product1 ==
  in_1 : Inport  Port=1  LatchInput=off
  in_2 : Inport  Port=2  LatchInput=off
  Product : Product  SaturateOnIntegerOverflow=on  RndMeth=Zero  InputSameDT=on
  Sum : Sum  Inputs=+  SaturateOnIntegerOverflow=on  InputSameDT=on
  out_1 : Outport  InitialOutput=0
  wires:
  in_2/1 -> Product/2
  in_1/1 -> Product/1
  Product/1 -> Sum/1
  Sum/1 -> out_1/1

== system rov_design_analysis/ROV Controller /Adaptive PD  Cascaded  Controller - 6 DoF/Body-fixed to Earth_fixed Transformation3/Transformation matrix R/Row3 of T/Dot Product1 ==
  in_1 : Inport  Port=1  LatchInput=off
  in_2 : Inport  Port=2  LatchInput=off
  Product : Product  SaturateOnIntegerOverflow=on  RndMeth=Zero  InputSameDT=on
  Sum : Sum  Inputs=+  SaturateOnIntegerOverflow=on  InputSameDT=on
  out_1 : Outport  InitialOutput=0
  wires:
  in_2/1 -> Product/2
  in_1/1 -> Product/1
  Product/1 -> Sum/1
  Sum/1 -> out_1/1

== system rov_design_analysis/ROV Controller /Adaptive PD  Cascaded  Controller - 6 DoF/Body-fixed to Earth_fixed Transformation3/Transformation matrix T/Row1 of R/Dot Product ==
  in_1 : Inport  Port=1  LatchInput=off
  in_2 : Inport  Port=2  LatchInput=off
  Product : Product  SaturateOnIntegerOverflow=on  RndMeth=Zero  InputSameDT=on
  Sum : Sum  Inputs=+  SaturateOnIntegerOverflow=on  InputSameDT=on
  out_1 : Outport  InitialOutput=0
  wires:
  in_2/1 -> Product/2
  in_1/1 -> Product/1
  Product/1 -> Sum/1
  Sum/1 -> out_1/1

== system rov_design_analysis/ROV Controller /Adaptive PD  Cascaded  Controller - 6 DoF/Body-fixed to Earth_fixed Transformation3/Transformation matrix T/Row2 of R/Dot Product1 ==
  in_1 : Inport  Port=1  LatchInput=off
  in_2 : Inport  Port=2  LatchInput=off
  Product : Product  SaturateOnIntegerOverflow=on  RndMeth=Zero  InputSameDT=on
  Sum : Sum  Inputs=+  SaturateOnIntegerOverflow=on  InputSameDT=on
  out_1 : Outport  InitialOutput=0
  wires:
  in_2/1 -> Product/2
  in_1/1 -> Product/1
  Product/1 -> Sum/1
  Sum/1 -> out_1/1

== system rov_design_analysis/ROV Controller /Adaptive PD  Cascaded  Controller - 6 DoF/Body-fixed to Earth_fixed Transformation3/Transformation matrix T/Row3 of R/Dot Product1 ==
  in_1 : Inport  Port=1  LatchInput=off
  in_2 : Inport  Port=2  LatchInput=off
  Product : Product  SaturateOnIntegerOverflow=on  RndMeth=Zero  InputSameDT=on
  Sum : Sum  Inputs=+  SaturateOnIntegerOverflow=on  InputSameDT=on
  out_1 : Outport  InitialOutput=0
  wires:
  in_2/1 -> Product/2
  in_1/1 -> Product/1
  Product/1 -> Sum/1
  Sum/1 -> out_1/1

== system rov_design_analysis/ROV Controller /Hybrid Control- one DoF/Body-fixed to Earth_fixed Transformation1/Transformation matrix R/Row1 of T/Dot Product1 ==
  in_1 : Inport  Port=1  LatchInput=off
  in_2 : Inport  Port=2  LatchInput=off
  Product : Product  SaturateOnIntegerOverflow=on  RndMeth=Zero  InputSameDT=on
  Sum : Sum  Inputs=+  SaturateOnIntegerOverflow=on  InputSameDT=on
  out_1 : Outport  InitialOutput=0
  wires:
  in_2/1 -> Product/2
  in_1/1 -> Product/1
  Product/1 -> Sum/1
  Sum/1 -> out_1/1

== system rov_design_analysis/ROV Controller /Hybrid Control- one DoF/Body-fixed to Earth_fixed Transformation1/Transformation matrix R/Row2 of T/Dot Product1 ==
  in_1 : Inport  Port=1  LatchInput=off
  in_2 : Inport  Port=2  LatchInput=off
  Product : Product  SaturateOnIntegerOverflow=on  RndMeth=Zero  InputSameDT=on
  Sum : Sum  Inputs=+  SaturateOnIntegerOverflow=on  InputSameDT=on
  out_1 : Outport  InitialOutput=0
  wires:
  in_2/1 -> Product/2
  in_1/1 -> Product/1
  Product/1 -> Sum/1
  Sum/1 -> out_1/1

== system rov_design_analysis/ROV Controller /Hybrid Control- one DoF/Body-fixed to Earth_fixed Transformation1/Transformation matrix R/Row3 of T/Dot Product1 ==
  in_1 : Inport  Port=1  LatchInput=off
  in_2 : Inport  Port=2  LatchInput=off
  Product : Product  SaturateOnIntegerOverflow=on  RndMeth=Zero  InputSameDT=on
  Sum : Sum  Inputs=+  SaturateOnIntegerOverflow=on  InputSameDT=on
  out_1 : Outport  InitialOutput=0
  wires:
  in_2/1 -> Product/2
  in_1/1 -> Product/1
  Product/1 -> Sum/1
  Sum/1 -> out_1/1

== system rov_design_analysis/ROV Controller /Hybrid Control- one DoF/Body-fixed to Earth_fixed Transformation1/Transformation matrix T/Row1 of R/Dot Product ==
  in_1 : Inport  Port=1  LatchInput=off
  in_2 : Inport  Port=2  LatchInput=off
  Product : Product  SaturateOnIntegerOverflow=on  RndMeth=Zero  InputSameDT=on
  Sum : Sum  Inputs=+  SaturateOnIntegerOverflow=on  InputSameDT=on
  out_1 : Outport  InitialOutput=0
  wires:
  in_2/1 -> Product/2
  in_1/1 -> Product/1
  Product/1 -> Sum/1
  Sum/1 -> out_1/1

== system rov_design_analysis/ROV Controller /Hybrid Control- one DoF/Body-fixed to Earth_fixed Transformation1/Transformation matrix T/Row2 of R/Dot Product1 ==
  in_1 : Inport  Port=1  LatchInput=off
  in_2 : Inport  Port=2  LatchInput=off
  Product : Product  SaturateOnIntegerOverflow=on  RndMeth=Zero  InputSameDT=on
  Sum : Sum  Inputs=+  SaturateOnIntegerOverflow=on  InputSameDT=on
  out_1 : Outport  InitialOutput=0
  wires:
  in_2/1 -> Product/2
  in_1/1 -> Product/1
  Product/1 -> Sum/1
  Sum/1 -> out_1/1

== system rov_design_analysis/ROV Controller /Hybrid Control- one DoF/Body-fixed to Earth_fixed Transformation1/Transformation matrix T/Row3 of R/Dot Product1 ==
  in_1 : Inport  Port=1  LatchInput=off
  in_2 : Inport  Port=2  LatchInput=off
  Product : Product  SaturateOnIntegerOverflow=on  RndMeth=Zero  InputSameDT=on
  Sum : Sum  Inputs=+  SaturateOnIntegerOverflow=on  InputSameDT=on
  out_1 : Outport  InitialOutput=0
  wires:
  in_2/1 -> Product/2
  in_1/1 -> Product/1
  Product/1 -> Sum/1
  Sum/1 -> out_1/1

== system rov_design_analysis/ROV Controller /Hybrid Control- one DoF/Body-fixed to Earth_fixed Transformation3/Transformation matrix R/Row1 of T/Dot Product1 ==
  in_1 : Inport  Port=1  LatchInput=off
  in_2 : Inport  Port=2  LatchInput=off
  Product : Product  SaturateOnIntegerOverflow=on  RndMeth=Zero  InputSameDT=on
  Sum : Sum  Inputs=+  SaturateOnIntegerOverflow=on  InputSameDT=on
  out_1 : Outport  InitialOutput=0
  wires:
  Sum/1 -> out_1/1
  Product/1 -> Sum/1
  in_1/1 -> Product/1
  in_2/1 -> Product/2

== system rov_design_analysis/ROV Controller /Hybrid Control- one DoF/Body-fixed to Earth_fixed Transformation3/Transformation matrix R/Row2 of T/Dot Product1 ==
  in_1 : Inport  Port=1  LatchInput=off
  in_2 : Inport  Port=2  LatchInput=off
  Product : Product  SaturateOnIntegerOverflow=on  RndMeth=Zero  InputSameDT=on
  Sum : Sum  Inputs=+  SaturateOnIntegerOverflow=on  InputSameDT=on
  out_1 : Outport  InitialOutput=0
  wires:
  Sum/1 -> out_1/1
  Product/1 -> Sum/1
  in_1/1 -> Product/1
  in_2/1 -> Product/2

== system rov_design_analysis/ROV Controller /Hybrid Control- one DoF/Body-fixed to Earth_fixed Transformation3/Transformation matrix R/Row3 of T/Dot Product1 ==
  in_1 : Inport  Port=1  LatchInput=off
  in_2 : Inport  Port=2  LatchInput=off
  Product : Product  SaturateOnIntegerOverflow=on  RndMeth=Zero  InputSameDT=on
  Sum : Sum  Inputs=+  SaturateOnIntegerOverflow=on  InputSameDT=on
  out_1 : Outport  InitialOutput=0
  wires:
  Sum/1 -> out_1/1
  Product/1 -> Sum/1
  in_1/1 -> Product/1
  in_2/1 -> Product/2

== system rov_design_analysis/ROV Controller /Hybrid Control- one DoF/Body-fixed to Earth_fixed Transformation3/Transformation matrix T/Row1 of R/Dot Product ==
  in_1 : Inport  Port=1  LatchInput=off
  in_2 : Inport  Port=2  LatchInput=off
  Product : Product  SaturateOnIntegerOverflow=on  RndMeth=Zero  InputSameDT=on
  Sum : Sum  Inputs=+  SaturateOnIntegerOverflow=on  InputSameDT=on
  out_1 : Outport  InitialOutput=0
  wires:
  Sum/1 -> out_1/1
  Product/1 -> Sum/1
  in_1/1 -> Product/1
  in_2/1 -> Product/2

== system rov_design_analysis/ROV Controller /Hybrid Control- one DoF/Body-fixed to Earth_fixed Transformation3/Transformation matrix T/Row2 of R/Dot Product1 ==
  in_1 : Inport  Port=1  LatchInput=off
  in_2 : Inport  Port=2  LatchInput=off
  Product : Product  SaturateOnIntegerOverflow=on  RndMeth=Zero  InputSameDT=on
  Sum : Sum  Inputs=+  SaturateOnIntegerOverflow=on  InputSameDT=on
  out_1 : Outport  InitialOutput=0
  wires:
  Sum/1 -> out_1/1
  Product/1 -> Sum/1
  in_1/1 -> Product/1
  in_2/1 -> Product/2

== system rov_design_analysis/ROV Controller /Hybrid Control- one DoF/Body-fixed to Earth_fixed Transformation3/Transformation matrix T/Row3 of R/Dot Product1 ==
  in_1 : Inport  Port=1  LatchInput=off
  in_2 : Inport  Port=2  LatchInput=off
  Product : Product  SaturateOnIntegerOverflow=on  RndMeth=Zero  InputSameDT=on
  Sum : Sum  Inputs=+  SaturateOnIntegerOverflow=on  InputSameDT=on
  out_1 : Outport  InitialOutput=0
  wires:
  Sum/1 -> out_1/1
  Product/1 -> Sum/1
  in_1/1 -> Product/1
  in_2/1 -> Product/2

== system rov_design_analysis/ROV Controller /Nonlinear-Based PD  Cascaded  Controller - 6 DoF/Body-fixed to Earth_fixed Transformation1/Transformation matrix R/Row1 of T/Dot Product1 ==
  in_1 : Inport  Port=1  LatchInput=off
  in_2 : Inport  Port=2  LatchInput=off
  Product : Product  SaturateOnIntegerOverflow=on  RndMeth=Zero  InputSameDT=on
  Sum : Sum  Inputs=+  SaturateOnIntegerOverflow=on  InputSameDT=on
  out_1 : Outport  InitialOutput=0
  wires:
  in_2/1 -> Product/2
  in_1/1 -> Product/1
  Product/1 -> Sum/1
  Sum/1 -> out_1/1

== system rov_design_analysis/ROV Controller /Nonlinear-Based PD  Cascaded  Controller - 6 DoF/Body-fixed to Earth_fixed Transformation1/Transformation matrix R/Row2 of T/Dot Product1 ==
  in_1 : Inport  Port=1  LatchInput=off
  in_2 : Inport  Port=2  LatchInput=off
  Product : Product  SaturateOnIntegerOverflow=on  RndMeth=Zero  InputSameDT=on
  Sum : Sum  Inputs=+  SaturateOnIntegerOverflow=on  InputSameDT=on
  out_1 : Outport  InitialOutput=0
  wires:
  in_2/1 -> Product/2
  in_1/1 -> Product/1
  Product/1 -> Sum/1
  Sum/1 -> out_1/1

== system rov_design_analysis/ROV Controller /Nonlinear-Based PD  Cascaded  Controller - 6 DoF/Body-fixed to Earth_fixed Transformation1/Transformation matrix R/Row3 of T/Dot Product1 ==
  in_1 : Inport  Port=1  LatchInput=off
  in_2 : Inport  Port=2  LatchInput=off
  Product : Product  SaturateOnIntegerOverflow=on  RndMeth=Zero  InputSameDT=on
  Sum : Sum  Inputs=+  SaturateOnIntegerOverflow=on  InputSameDT=on
  out_1 : Outport  InitialOutput=0
  wires:
  in_2/1 -> Product/2
  in_1/1 -> Product/1
  Product/1 -> Sum/1
  Sum/1 -> out_1/1

== system rov_design_analysis/ROV Controller /Nonlinear-Based PD  Cascaded  Controller - 6 DoF/Body-fixed to Earth_fixed Transformation1/Transformation matrix T/Row1 of R/Dot Product ==
  in_1 : Inport  Port=1  LatchInput=off
  in_2 : Inport  Port=2  LatchInput=off
  Product : Product  SaturateOnIntegerOverflow=on  RndMeth=Zero  InputSameDT=on
  Sum : Sum  Inputs=+  SaturateOnIntegerOverflow=on  InputSameDT=on
  out_1 : Outport  InitialOutput=0
  wires:
  in_2/1 -> Product/2
  in_1/1 -> Product/1
  Product/1 -> Sum/1
  Sum/1 -> out_1/1

== system rov_design_analysis/ROV Controller /Nonlinear-Based PD  Cascaded  Controller - 6 DoF/Body-fixed to Earth_fixed Transformation1/Transformation matrix T/Row2 of R/Dot Product1 ==
  in_1 : Inport  Port=1  LatchInput=off
  in_2 : Inport  Port=2  LatchInput=off
  Product : Product  SaturateOnIntegerOverflow=on  RndMeth=Zero  InputSameDT=on
  Sum : Sum  Inputs=+  SaturateOnIntegerOverflow=on  InputSameDT=on
  out_1 : Outport  InitialOutput=0
  wires:
  in_2/1 -> Product/2
  in_1/1 -> Product/1
  Product/1 -> Sum/1
  Sum/1 -> out_1/1

== system rov_design_analysis/ROV Controller /Nonlinear-Based PD  Cascaded  Controller - 6 DoF/Body-fixed to Earth_fixed Transformation1/Transformation matrix T/Row3 of R/Dot Product1 ==
  in_1 : Inport  Port=1  LatchInput=off
  in_2 : Inport  Port=2  LatchInput=off
  Product : Product  SaturateOnIntegerOverflow=on  RndMeth=Zero  InputSameDT=on
  Sum : Sum  Inputs=+  SaturateOnIntegerOverflow=on  InputSameDT=on
  out_1 : Outport  InitialOutput=0
  wires:
  in_2/1 -> Product/2
  in_1/1 -> Product/1
  Product/1 -> Sum/1
  Sum/1 -> out_1/1

== system rov_design_analysis/ROV Controller /Nonlinear-Based PD  Cascaded  Controller - 6 DoF/Body-fixed to Earth_fixed Transformation3/Transformation matrix R/Row1 of T/Dot Product1 ==
  in_1 : Inport  Port=1  LatchInput=off
  in_2 : Inport  Port=2  LatchInput=off
  Product : Product  SaturateOnIntegerOverflow=on  RndMeth=Zero  InputSameDT=on
  Sum : Sum  Inputs=+  SaturateOnIntegerOverflow=on  InputSameDT=on
  out_1 : Outport  InitialOutput=0
  wires:
  Sum/1 -> out_1/1
  Product/1 -> Sum/1
  in_1/1 -> Product/1
  in_2/1 -> Product/2

== system rov_design_analysis/ROV Controller /Nonlinear-Based PD  Cascaded  Controller - 6 DoF/Body-fixed to Earth_fixed Transformation3/Transformation matrix R/Row2 of T/Dot Product1 ==
  in_1 : Inport  Port=1  LatchInput=off
  in_2 : Inport  Port=2  LatchInput=off
  Product : Product  SaturateOnIntegerOverflow=on  RndMeth=Zero  InputSameDT=on
  Sum : Sum  Inputs=+  SaturateOnIntegerOverflow=on  InputSameDT=on
  out_1 : Outport  InitialOutput=0
  wires:
  Sum/1 -> out_1/1
  Product/1 -> Sum/1
  in_1/1 -> Product/1
  in_2/1 -> Product/2

== system rov_design_analysis/ROV Controller /Nonlinear-Based PD  Cascaded  Controller - 6 DoF/Body-fixed to Earth_fixed Transformation3/Transformation matrix R/Row3 of T/Dot Product1 ==
  in_1 : Inport  Port=1  LatchInput=off
  in_2 : Inport  Port=2  LatchInput=off
  Product : Product  SaturateOnIntegerOverflow=on  RndMeth=Zero  InputSameDT=on
  Sum : Sum  Inputs=+  SaturateOnIntegerOverflow=on  InputSameDT=on
  out_1 : Outport  InitialOutput=0
  wires:
  Sum/1 -> out_1/1
  Product/1 -> Sum/1
  in_1/1 -> Product/1
  in_2/1 -> Product/2

== system rov_design_analysis/ROV Controller /Nonlinear-Based PD  Cascaded  Controller - 6 DoF/Body-fixed to Earth_fixed Transformation3/Transformation matrix T/Row1 of R/Dot Product ==
  in_1 : Inport  Port=1  LatchInput=off
  in_2 : Inport  Port=2  LatchInput=off
  Product : Product  SaturateOnIntegerOverflow=on  RndMeth=Zero  InputSameDT=on
  Sum : Sum  Inputs=+  SaturateOnIntegerOverflow=on  InputSameDT=on
  out_1 : Outport  InitialOutput=0
  wires:
  Sum/1 -> out_1/1
  Product/1 -> Sum/1
  in_1/1 -> Product/1
  in_2/1 -> Product/2

== system rov_design_analysis/ROV Controller /Nonlinear-Based PD  Cascaded  Controller - 6 DoF/Body-fixed to Earth_fixed Transformation3/Transformation matrix T/Row2 of R/Dot Product1 ==
  in_1 : Inport  Port=1  LatchInput=off
  in_2 : Inport  Port=2  LatchInput=off
  Product : Product  SaturateOnIntegerOverflow=on  RndMeth=Zero  InputSameDT=on
  Sum : Sum  Inputs=+  SaturateOnIntegerOverflow=on  InputSameDT=on
  out_1 : Outport  InitialOutput=0
  wires:
  Sum/1 -> out_1/1
  Product/1 -> Sum/1
  in_1/1 -> Product/1
  in_2/1 -> Product/2

== system rov_design_analysis/ROV Controller /Nonlinear-Based PD  Cascaded  Controller - 6 DoF/Body-fixed to Earth_fixed Transformation3/Transformation matrix T/Row3 of R/Dot Product1 ==
  in_1 : Inport  Port=1  LatchInput=off
  in_2 : Inport  Port=2  LatchInput=off
  Product : Product  SaturateOnIntegerOverflow=on  RndMeth=Zero  InputSameDT=on
  Sum : Sum  Inputs=+  SaturateOnIntegerOverflow=on  InputSameDT=on
  out_1 : Outport  InitialOutput=0
  wires:
  Sum/1 -> out_1/1
  Product/1 -> Sum/1
  in_1/1 -> Product/1
  in_2/1 -> Product/2

== system rov_design_analysis/ROV Controller /Nonlinear-Sliding-Mode Cascaded  Controller - 6 DoF/Body-fixed to Earth_fixed Transformation1/Transformation matrix R/Row1 of T/Dot Product1 ==
  in_1 : Inport  Port=1  LatchInput=off
  in_2 : Inport  Port=2  LatchInput=off
  Product : Product  SaturateOnIntegerOverflow=on  RndMeth=Zero  InputSameDT=on
  Sum : Sum  Inputs=+  SaturateOnIntegerOverflow=on  InputSameDT=on
  out_1 : Outport  InitialOutput=0
  wires:
  Sum/1 -> out_1/1
  Product/1 -> Sum/1
  in_1/1 -> Product/1
  in_2/1 -> Product/2
